simulink model "SP_OEL2"  (R2023b)
settings: Solver=ode23t  StartTime=0.0  StopTime=0.6  MaxStep=simulation.maxStepSize  RelTol=1e-3  AbsTol=1e-3
PostLoadFcn:
  | run('OCR_input.m');
  | run('OCR_settings.m');
InitFcn:
  | run('OCR_settings.m');
undefined symbols (not defined in the file or in its folder): relay1, relay2, source
libraries: ee_lib x14, fl_lib x8, eeGeneralControl x8, simulink x4, simulink_extras x4, nesl_utility x2
(part 1 of 2)
CloseFcn:
  | try, close(h1_ee_relay_overcurrent_phase), end
  | clear h1_ee_relay_overcurrent_phase
  | try, close(h2_ee_relay_overcurrent_earth), end
  | clear h2_ee_relay_overcurrent_earth
  | clear source;
  | clear transformer;
  | clear distributionLine1;
  | clear distributionLine2;
  | clear load;
  | clear sensor1;
  | clear sensor2;
  | clear fault;
  | clear protection;
  | clear maskParameter;
  | clear simlog_ee_relay_overcurrent_protection;
  | clear simulation;
  | clear relay1;
  | clear relay2;
  | clear plotVar;
  | clear relayType;
  | clear mask;
Description:
  | Overcurrent Relay Protection in AC Microgrid
settings Model: Creator=The MathWorks, Inc.  LastModifiedBy=hazwani
settings SolverCC: MaxConsecutiveZCs=100000  MaxConsecutiveMinStep=1000  MaxZcPerStep=1
settings DataIOCC: SaveOutput=off  SignalLogging=off  DSMLogging=off  SaveTime=off  ReturnWorkspaceOutputs=off
settings OptimizationCC: ReuseModelBlockBuffer=off
settings DebuggingCC: UnconnectedInputMsg=warning  UnconnectedOutputMsg=warning  UnconnectedLineMsg=warning
settings ModelReferenceCC: EnableRefExpFcnMdlSchedulingChecks=on
settings RTWCC: DLArmComputeVersion=19.05
settings SimscapeCC: SimscapeLogType=all  SimscapeLogName=simlog_ee_relay_overcurrent_protection  SimscapeLogLimitData=off

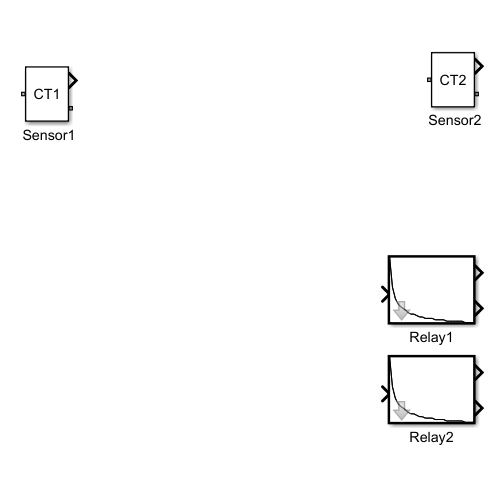
[thumbnail: Simulink's stored preview of the top-level diagram]
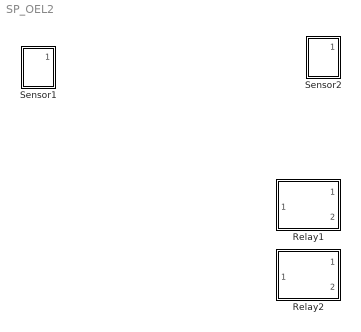
== system SP_OEL2 ==
  " Sensor1" : Subsystem
      mask Display: disp('CT1')
  " Sensor2" : Subsystem
      mask Display: disp('CT2')
  Relay1 : Subsystem  TreatAsAtomicUnit=on  SystemSampleTime=relay1.sampleTime  mask{relayCharacteristicPhase=IEEE Moderately Inverse, relayCharacteristicEarth=IEEE Moderately Inverse, ratedFrequency=source.ratedFrequency, sampleTime=relay1.sampleTime, protectionEnable=1, currentPhase=[1.5 2.5 3.5 4.5 5.5 6.5 7.5 8.5 9.5 10.5], tmsPhase=[0.1 0.2], topPhase=[0.64 1.29;0.29 0.58;0.21 0.43;0.18 0.36;0.16 0.32;0.15 0.29;0.14 0.27;0.13 0.26;0.12 0.25;0.12 0.24], currentEarth=[0.06 0.15 0.2 0.25 0.3 0.35 0.4 0.45 0.5 0.55], tmsEarth=[0.1 0.2], topEarth=[0.64 1.29;0.29 0.58;0.21 0.43;0.18 0.36;0.16 0.32;0.15 0.29;0.14 0.27;0.13 0.26;0.12 0.25;0.12 0.24], phPickUp=relay1.phFltPickUp, ethPickUp=relay1.erFltPickUp, phTimeSetting=relay1.phFltTMS, ethTimeSetting=relay1.erFltTMS, topPhaseActual=0.2, topEarthActual=0.3}
      mask prompts: relayCharacteristicPhase "Relay characteristics for phase protection"; relayCharacteristicEarth "Relay characteristics for earth protection"; ratedFrequency "Fundamental frequency (Hz)"; sampleTime "Relay sample time (s)"; protectionEnable "Relay operation enable"; currentPhase "Current setting for phase protection (A)"; tmsPhase "Time multiplier setting for phase protection (s)"; topPhase "Operating time for phase protection (s)"; currentEarth "Current setting for earth protection (A)"; tmsEarth "Time multiplier setting for earth protection (s)"; topEarth "Operating time for earth protection (s)"; phPickUp "Pick up current for phase protection (A)"; ethPickUp "Pick up current for earth protection (A)"; phTimeSetting "Time multiplier setting for phase protection (s)"; ethTimeSetting "Time multiplier setting for earth protection (s)"; topPhaseActual "Relay operating time for phase protection (s)"; topEarthActual "Relay operating time for earth protection (s)"
      mask TypeOptions relayCharacteristicPhase: IEC Normal Inverse | IEC Very Inverse | IEC Extremely Inverse | IEEE Moderately Inverse | IEEE Very Inverse | IEEE Extremely Inverse | Definite Time | IvsT
      mask Callback relayCharacteristicPhase:
      | % Control parameter visiblity
      | enablePhase = get_param(gcb,'relayCharacteristicPhase');
      | enableEarth = get_param(gcb,'relayCharacteristicEarth');
      | % Set the 'MaskVisibilities' property for each parameters
      | cArray=cell(1,17);
      | cArray(:)={'on'};
      | p=strcmp(enablePhase,'IvsT');
      | q=strcmp(enableEarth,'IvsT');
      | r=strcmp(enablePhase,'Definite Time');
      | s=strcmp(enableEarth,'Definite Time');
      | if p==0 && q==1
      |     cArray(6:8)={'off'};
      | elseif p==0 && q==0
      |     cArray(6:11)={'off'};
      | elseif p==1 && q==0
      |     cArray(9:11)={'off'};
      | end
      | if r==0 && s==1
      |     cArray(15)={'off'};
      |     cArray(16)={'off'};
      | elseif r==0 && s==0
      |     cArray(16:17)={'off'};
      | elseif r==1 && s==0
      |     cArray(14)={'off'};
      |     cArray(17)={'off'};
      | elseif r==1 && s==1
      |     cArray(14:15)={'off'};
      | end
      | set_param(gcb,'MaskVisibilities',cArray);
      mask TypeOptions relayCharacteristicEarth: IEC Normal Inverse | IEC Very Inverse | IEC Extremely Inverse | IEEE Moderately Inverse | IEEE Very Inverse | IEEE Extremely Inverse | Definite Time | IvsT
      mask Callback relayCharacteristicEarth:
      | % Control parameter visiblity
      | enablePhase = get_param(gcb,'relayCharacteristicPhase');
      | enableEarth = get_param(gcb,'relayCharacteristicEarth');
      | % Set the 'MaskVisibilities' property for each parameters
      | cArray=cell(1,17);
      | cArray(:)={'on'};
      | p=strcmp(enablePhase,'IvsT');
      | q=strcmp(enableEarth,'IvsT');
      | r=strcmp(enablePhase,'Definite Time');
      | s=strcmp(enableEarth,'Definite Time');
      | if p==0 && q==1
      |     cArray(6:8)={'off'};
      | elseif p==0 && q==0
      |     cArray(6:11)={'off'};
      | elseif p==1 && q==0
      |     cArray(9:11)={'off'};
      | end
      | if r==0 && s==1
      |     cArray(15)={'off'};
      |     cArray(16)={'off'};
      | elseif r==0 && s==0
      |     cArray(16:17)={'off'};
      | elseif r==1 && s==0
      |     cArray(14)={'off'};
      |     cArray(17)={'off'};
      | elseif r==1 && s==1
      |     cArray(14:15)={'off'};
      | end
      | set_param(gcb,'MaskVisibilities',cArray);
      mask DialogControl Container9 Prompt: Main
      mask DialogControl Container24 Prompt: Current Settings
      mask DialogControl Container19 Prompt: Time Settings
      mask Display:
      | psm = 1:1:30; % Plug setting multiplier
      | tms=0.01; % Time multiplier setting is assumed to be 0.01s
      | top=ones(2,length(psm));  % Operating time of the relay
      | maskParameter=Simulink.Mask.get(gcb); % Get the mask parameters
      | for i=1:2
      |     index(i)=find(strcmp(maskParameter.Parameters(1,i).Value,maskParameter.Parameters(1,i).TypeOptions));
      |     if index(i)<7
      |         switch index(i)              % Selection of relay characteristic
      |             case 1                   % IEC Normal Inverse
      |                 a=0.14;
      |                 b=0.02;
      |                 c=0;
      |             case 2                   % IEC Very Inverse
      |                 a=13.5;
      |                 b=1;
      |                 c=0;
      |             case 3                   % IEC Extremely Inverse
      |                 a=80;
      |                 b=2;
      |                 c=0;
      |             case 4                   % IEEE Moderately Inverse
      |                 a=0.0515;
      |                 b=0.02;
      |                 c=0.114;
      |             case 5                   % IEEE Very Inverse
      |                 a=19.61;
      |                 b=2;
      |                 c=0.491;
      |             otherwise                % IEEE Exteremely Inverse
      |                 a=28.2;
      |                 b=2;
      |                 c=0.1217;
      |         end
      |         for j=1:length(psm)
      |             top(i,j)=tms*((a/(power(psm(j),b)-1))+c); % Operating time of the relay
      |         end
      |     else
      |         top(i,1:length(psm))=0.03*ones(1,length(psm));% Operating time of the relay
      |     end
      | end
      | top1=top(1,1:end);
      | top2=top(2,1:end);
      | 
      | maskFigure=figure;
      | if index(1)<8
      |     plot(psm,top1)
      | else
      |     fprintf('\n\nIvsT');
      | end
      | hold on;
      | if index(2)<8
      |     plot(psm,top2);
      | elseif index(1)<8
      |     fprintf('\nIvsT');
      | end
      | close(maskFigure);
  Relay2 : Subsystem  TreatAsAtomicUnit=on  SystemSampleTime=relay1.sampleTime  mask{relayCharacteristicPhase=IEEE Moderately Inverse, relayCharacteristicEarth=IEEE Moderately Inverse, ratedFrequency=source.ratedFrequency, sampleTime=relay2.sampleTime, protectionEnable=1, currentPhase=[1.5 2.5 3.5 4.5 5.5 6.5 7.5 8.5 9.5 10.5], tmsPhase=[0.1 0.2], topPhase=[0.64 1.29;0.29 0.58;0.21 0.43;0.18 0.36;0.16 0.32;0.15 0.29;0.14 0.27;0.13 0.26;0.12 0.25;0.12 0.24], currentEarth=[0.06 0.15 0.2 0.25 0.3 0.35 0.4 0.45 0.5 0.55], tmsEarth=[0.1 0.2], topEarth=[0.64 1.29;0.29 0.58;0.21 0.43;0.18 0.36;0.16 0.32;0.15 0.29;0.14 0.27;0.13 0.26;0.12 0.25;0.12 0.24], phPickUp=relay2.phFltPickUp, ethPickUp=relay2.erFltPickUp, phTimeSetting=relay2.phFltTMS, ethTimeSetting=relay2.erFltTMS, topPhaseActual=0.2, topEarthActual=0.3}
      mask prompts: relayCharacteristicPhase "Relay characteristics for phase protection"; relayCharacteristicEarth "Relay characteristics for earth protection"; ratedFrequency "Fundamental frequency (Hz)"; sampleTime "Relay sample time (s)"; protectionEnable "Relay operation enable"; currentPhase "Current setting for phase protection (A)"; tmsPhase "Time multiplier setting for phase protection (s)"; topPhase "Operating time for phase protection (s)"; currentEarth "Current setting for earth protection (A)"; tmsEarth "Time multiplier setting for earth protection (s)"; topEarth "Operating time for earth protection (s)"; phPickUp "Pick up current for phase protection (A)"; ethPickUp "Pick up current for earth protection (A)"; phTimeSetting "Time multiplier setting for phase protection (s)"; ethTimeSetting "Time multiplier setting for earth protection (s)"; topPhaseActual "Relay operating time for phase protection (s)"; topEarthActual "Relay operating time for earth protection (s)"
      mask TypeOptions relayCharacteristicPhase: IEC Normal Inverse | IEC Very Inverse | IEC Extremely Inverse | IEEE Moderately Inverse | IEEE Very Inverse | IEEE Extremely Inverse | Definite Time | IvsT
      mask Callback relayCharacteristicPhase:
      | % Control parameter visiblity
      | enablePhase = get_param(gcb,'relayCharacteristicPhase');
      | enableEarth = get_param(gcb,'relayCharacteristicEarth');
      | % Set the 'MaskVisibilities' property for each parameters
      | cArray=cell(1,17);
      | cArray(:)={'on'};
      | p=strcmp(enablePhase,'IvsT');
      | q=strcmp(enableEarth,'IvsT');
      | r=strcmp(enablePhase,'Definite Time');
      | s=strcmp(enableEarth,'Definite Time');
      | if p==0 && q==1
      |     cArray(6:8)={'off'};
      | elseif p==0 && q==0
      |     cArray(6:11)={'off'};
      | elseif p==1 && q==0
      |     cArray(9:11)={'off'};
      | end
      | if r==0 && s==1
      |     cArray(15)={'off'};
      |     cArray(16)={'off'};
      | elseif r==0 && s==0
      |     cArray(16:17)={'off'};
      | elseif r==1 && s==0
      |     cArray(14)={'off'};
      |     cArray(17)={'off'};
      | elseif r==1 && s==1
      |     cArray(14:15)={'off'};
      | end
      | set_param(gcb,'MaskVisibilities',cArray);
      mask TypeOptions relayCharacteristicEarth: IEC Normal Inverse | IEC Very Inverse | IEC Extremely Inverse | IEEE Moderately Inverse | IEEE Very Inverse | IEEE Extremely Inverse | Definite Time | IvsT
      mask Callback relayCharacteristicEarth:
      | % Control parameter visiblity
      | enablePhase = get_param(gcb,'relayCharacteristicPhase');
      | enableEarth = get_param(gcb,'relayCharacteristicEarth');
      | % Set the 'MaskVisibilities' property for each parameters
      | cArray=cell(1,17);
      | cArray(:)={'on'};
      | p=strcmp(enablePhase,'IvsT');
      | q=strcmp(enableEarth,'IvsT');
      | r=strcmp(enablePhase,'Definite Time');
      | s=strcmp(enableEarth,'Definite Time');
      | if p==0 && q==1
      |     cArray(6:8)={'off'};
      | elseif p==0 && q==0
      |     cArray(6:11)={'off'};
      | elseif p==1 && q==0
      |     cArray(9:11)={'off'};
      | end
      | if r==0 && s==1
      |     cArray(15)={'off'};
      |     cArray(16)={'off'};
      | elseif r==0 && s==0
      |     cArray(16:17)={'off'};
      | elseif r==1 && s==0
      |     cArray(14)={'off'};
      |     cArray(17)={'off'};
      | elseif r==1 && s==1
      |     cArray(14:15)={'off'};
      | end
      | set_param(gcb,'MaskVisibilities',cArray);
      mask DialogControl Container9 Prompt: Main
      mask DialogControl Container24 Prompt: Current Settings
      mask DialogControl Container19 Prompt: Time Settings
      mask Display:
      | psm = 1:1:30; % Plug setting multiplier
      | tms=0.01; % Time multiplier setting is assumed to be 0.01s
      | top=ones(2,length(psm));  % Operating time of the relay
      | maskParameter=Simulink.Mask.get(gcb); % Get the mask parameters
      | for i=1:2
      |     index(i)=find(strcmp(maskParameter.Parameters(1,i).Value,maskParameter.Parameters(1,i).TypeOptions));
      |     if index(i)<7
      |         switch index(i)              % Selection of relay characteristic
      |             case 1                   % IEC Normal Inverse
      |                 a=0.14;
      |                 b=0.02;
      |                 c=0;
      |             case 2                   % IEC Very Inverse
      |                 a=13.5;
      |                 b=1;
      |                 c=0;
      |             case 3                   % IEC Extremely Inverse
      |                 a=80;
      |                 b=2;
      |                 c=0;
      |             case 4                   % IEEE Moderately Inverse
      |                 a=0.0515;
      |                 b=0.02;
      |                 c=0.114;
      |             case 5                   % IEEE Very Inverse
      |                 a=19.61;
      |                 b=2;
      |                 c=0.491;
      |             otherwise                % IEEE Exteremely Inverse
      |                 a=28.2;
      |                 b=2;
      |                 c=0.1217;
      |         end
      |         for j=1:length(psm)
      |             top(i,j)=tms*((a/(power(psm(j),b)-1))+c); % Operating time of the relay
      |         end
      |     else
      |         top(i,1:length(psm))=0.03*ones(1,length(psm));% Operating time of the relay
      |     end
      | end
      | top1=top(1,1:end);
      | top2=top(2,1:end);
      | 
      | maskFigure=figure;
      | if index(1)<8
      |     plot(psm,top1)
      | else
      |     fprintf('\n\nIvsT');
      | end
      | hold on;
      | if index(2)<8
      |     plot(psm,top2);
      | elseif index(1)<8
      |     fprintf('\nIvsT');
      | end
      | close(maskFigure);

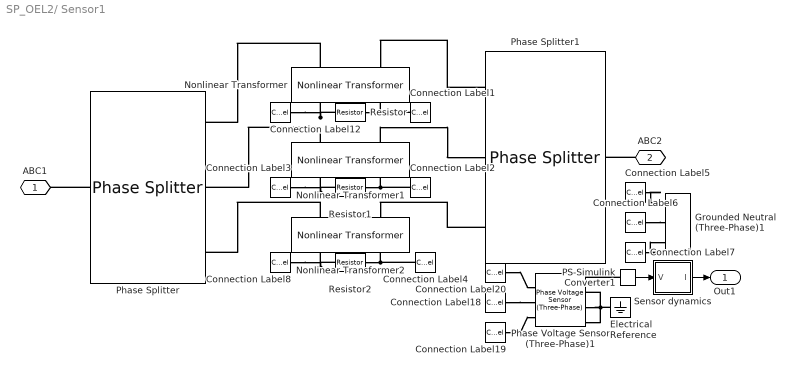
== system SP_OEL2/ Sensor1 ==
  Connection Label1 : ConnectionLabel  Label=Ian
  Connection Label12 : ConnectionLabel  Label=Iap
  Connection Label18 : ConnectionLabel  Label=Ibp
  Connection Label19 : ConnectionLabel  Label=Icp
  Connection Label2 : ConnectionLabel  Label=Ibn
  Connection Label20 : ConnectionLabel  Label=Iap
  Connection Label3 : ConnectionLabel  Label=Ibp
  Connection Label4 : ConnectionLabel  Label=Ibn
  Connection Label5 : ConnectionLabel  Label=Ian
  Connection Label6 : ConnectionLabel  Label=Ibn
  Connection Label7 : ConnectionLabel  Label=Icn
  Connection Label8 : ConnectionLabel  Label=Icp
  Electrical Reference : fl_lib/Electrical/Electrical Elements/Electrical Reference
  Grounded Neutral (Three-Phase)1 : ee_lib/Connectors & References/Grounded Neutral (Three-Phase)
      settings: InternalSimscapePortConfiguration="{\"Bottom\":[],\"Left\":[{\"id\":\"a\",\"label\":\"a\",\"type\":\"foundation.electrical.electrical\"},{\"id\":\"b\",\"label\":\"b\",\"type\":\"foundation.electrical.electrical\"},{\"id\":\"c\",\"label\":\"c\",\"type\":\"foundation.electrical.electrical\"}],\"Right\":[],\"Top\":[]}"
  Nonlinear Transformer : ee_lib/Passive/Transformers/Nonlinear Transformer  Nw=1  Nw2=sensor1.ctRatio  winding_param_option=1  Req=1e-3 Ohm  Leq=1e-4 H  R_1=0.01 Ohm  L_1=0.0001 H  R_2=0.01 Ohm  L_2=0.0001 H  averaging_period=0 s  R_m=100 Ohm  parameterization_option=1  H_data=[0, 200, 400, 600, 800, 1000] A/m  B_data=[0, .81, 1.25, 1.42, 1.48, 1.49] T  length_effective=0.2 m  area_effective=2e-4 m^2  L=4e-2 H  L_sat=1e-2 H  current_data=[0, .4, .8, 1.2, 1.6, 2] A  magnetic_flux_data=[0, .161, .25, .284, .295, .299] .* 1e-3 Wb  magnetic_flux_sat=1.6e-04 Wb  dBdH0=0.005 m*T/A  B1=1.49 T  H1=1000 A/m  c=0.1  K=200 A/m  alpha=1e-4  interpolation_option=1  Leq_i0=0 A  L1_i0=0 A  L2_i0=0 A  x0_option=1  i_L0=0 A  phi0=0 Wb  B0=0 T  H0=0 A/m  Leq_g=1e-9 1/Ohm  L1_g=1e-9 1/Ohm  L2_g=1e-9 1/Ohm
      settings: InternalSimscapePortConfiguration="{\"Bottom\":[],\"Left\":[{\"id\":\"p1\",\"label\":\"1+\",\"type\":\"foundation.electrical.electrical\"},{\"id\":\"n1\",\"label\":\"1-\",\"type\":\"foundation.electrical.electrical\"}],\"Right\":[{\"id\":\"p2\",\"label\":\"2+\",\"type\":\"foundation.electrical.electrical\"},{\"id\":\"n2\",\"label\":\"2-\",\"type\":\"foundation.electrical.electrical\"}],\"Top\":[]}"
  Nonlinear Transformer1 : ee_lib/Passive/Transformers/Nonlinear Transformer  Nw=1  Nw2=sensor1.ctRatio  winding_param_option=1  Req=1e-3 Ohm  Leq=1e-4 H  R_1=0.01 Ohm  L_1=0.0001 H  R_2=0.01 Ohm  L_2=0.0001 H  averaging_period=0 s  R_m=100 Ohm  parameterization_option=1  H_data=[0, 200, 400, 600, 800, 1000] A/m  B_data=[0, .81, 1.25, 1.42, 1.48, 1.49] T  length_effective=0.2 m  area_effective=2e-4 m^2  L=4e-2 H  L_sat=1e-2 H  current_data=[0, .4, .8, 1.2, 1.6, 2] A  magnetic_flux_data=[0, .161, .25, .284, .295, .299] .* 1e-3 Wb  magnetic_flux_sat=1.6e-04 Wb  dBdH0=0.005 m*T/A  B1=1.49 T  H1=1000 A/m  c=0.1  K=200 A/m  alpha=1e-4  interpolation_option=1  Leq_i0=0 A  L1_i0=0 A  L2_i0=0 A  x0_option=1  i_L0=0 A  phi0=0 Wb  B0=0 T  H0=0 A/m  Leq_g=1e-9 1/Ohm  L1_g=1e-9 1/Ohm  L2_g=1e-9 1/Ohm
      settings: InternalSimscapePortConfiguration="{\"Bottom\":[],\"Left\":[{\"id\":\"p1\",\"label\":\"1+\",\"type\":\"foundation.electrical.electrical\"},{\"id\":\"n1\",\"label\":\"1-\",\"type\":\"foundation.electrical.electrical\"}],\"Right\":[{\"id\":\"p2\",\"label\":\"2+\",\"type\":\"foundation.electrical.electrical\"},{\"id\":\"n2\",\"label\":\"2-\",\"type\":\"foundation.electrical.electrical\"}],\"Top\":[]}"
  Nonlinear Transformer2 : ee_lib/Passive/Transformers/Nonlinear Transformer  Nw=1  Nw2=sensor1.ctRatio  winding_param_option=1  Req=1e-3 Ohm  Leq=1e-4 H  R_1=0.01 Ohm  L_1=0.0001 H  R_2=0.01 Ohm  L_2=0.0001 H  averaging_period=0 s  R_m=100 Ohm  parameterization_option=1  H_data=[0, 200, 400, 600, 800, 1000] A/m  B_data=[0, .81, 1.25, 1.42, 1.48, 1.49] T  length_effective=0.2 m  area_effective=2e-4 m^2  L=4e-2 H  L_sat=1e-2 H  current_data=[0, .4, .8, 1.2, 1.6, 2] A  magnetic_flux_data=[0, .161, .25, .284, .295, .299] .* 1e-3 Wb  magnetic_flux_sat=1.6e-04 Wb  dBdH0=0.005 m*T/A  B1=1.49 T  H1=1000 A/m  c=0.1  K=200 A/m  alpha=1e-4  interpolation_option=1  Leq_i0=0 A  L1_i0=0 A  L2_i0=0 A  x0_option=1  i_L0=0 A  phi0=0 Wb  B0=0 T  H0=0 A/m  Leq_g=1e-9 1/Ohm  L1_g=1e-9 1/Ohm  L2_g=1e-9 1/Ohm
      settings: InternalSimscapePortConfiguration="{\"Bottom\":[],\"Left\":[{\"id\":\"p1\",\"label\":\"1+\",\"type\":\"foundation.electrical.electrical\"},{\"id\":\"n1\",\"label\":\"1-\",\"type\":\"foundation.electrical.electrical\"}],\"Right\":[{\"id\":\"p2\",\"label\":\"2+\",\"type\":\"foundation.electrical.electrical\"},{\"id\":\"n2\",\"label\":\"2-\",\"type\":\"foundation.electrical.electrical\"}],\"Top\":[]}"
  PS-Simulink Converter1 : nesl_utility/PS-Simulink Converter  PhysicalDomain=network_engine_domain  SubClassName=ps_output  LeftPortType=input  RightPortType=output  PseudoPeriodic=off  Frequencies=[]  VectorFormat=1-D array  Unit=inherit  AffineConversion=off
  Phase Splitter : ee_lib/Connectors & References/Phase Splitter
  Phase Splitter1 : ee_lib/Connectors & References/Phase Splitter
  Phase Voltage Sensor (Three-Phase)1 : ee_lib/Sensors & Transducers/Phase Voltage Sensor (Three-Phase)
      settings: LogSimulationData=on  InternalSimscapePortConfiguration="{\"Bottom\":[],\"Left\":[{\"id\":\"a1\",\"label\":\"a1\",\"type\":\"foundation.electrical.electrical\"},{\"id\":\"b1\",\"label\":\"b1\",\"type\":\"foundation.electrical.electrical\"},{\"id\":\"c1\",\"label\":\"c1\",\"type\":\"foundation.electrical.electrical\"}],\"Right\":[{\"id\":\"V_output\",\"label\":\"V\",\"type\":\"output\"},{\"id\":\"a2\",\"label\":\"a2\",\"type\":\"foundation.electrical.electrical\"},{\"id\":\"b2\",\"label\":\"b2\",\"type\":\"foundation.electrical.electrical\"},{\"id\":\"c2\",\"label\":\"c2\",\"type\":\"foundation.electrical.electrical\"}],\"Top\":[]}"
  Resistor : fl_lib/Electrical/Electrical Elements/Resistor  R=1 Ohm  i_specify=off  i_priority=None  i=0 A  i_nominal_specify=off  i_nominal_unit=A  i_nominal_value=1  v_specify=off  v_priority=None  v=0 V  v_nominal_specify=off  v_nominal_unit=V  v_nominal_value=1
  Resistor1 : fl_lib/Electrical/Electrical Elements/Resistor  R=1 Ohm  i_specify=off  i_priority=None  i=0 A  i_nominal_specify=off  i_nominal_unit=A  i_nominal_value=1  v_specify=off  v_priority=None  v=0 V  v_nominal_specify=off  v_nominal_unit=V  v_nominal_value=1
  Resistor2 : fl_lib/Electrical/Electrical Elements/Resistor  R=1 Ohm  i_specify=off  i_priority=None  i=0 A  i_nominal_specify=off  i_nominal_unit=A  i_nominal_value=1  v_specify=off  v_priority=None  v=0 V  v_nominal_specify=off  v_nominal_unit=V  v_nominal_value=1
  Sensor dynamics : Subsystem
  ABC1 : PMIOPort  Side=Left
  ABC2 : PMIOPort  Port=2  Side=Right
  Out1 : Outport
  wires:
  PS-Simulink Converter1/1 -> Sensor dynamics/1(V)
  Sensor dynamics/1(I) -> Out1/1
  connections:
  Phase Splitter/LConn1 -- ABC1/RConn1
  ABC2/RConn1 -- Phase Splitter1/LConn1
  Connection Label19/LConn1 -- Phase Voltage Sensor (Three-Phase)1/LConn3
  Connection Label18/LConn1 -- Phase Voltage Sensor (Three-Phase)1/LConn2
  PS-Simulink Converter1/LConn1 -- Phase Voltage Sensor (Three-Phase)1/RConn1
  Connection Label20/LConn1 -- Phase Voltage Sensor (Three-Phase)1/LConn1
  Nonlinear Transformer/RConn1 -- Resistor/LConn1 -- Connection Label12/LConn1
  Nonlinear Transformer/LConn1 -- Phase Splitter/RConn1
  Phase Splitter1/RConn1 -- Nonlinear Transformer/LConn2
  Resistor/RConn1 -- Connection Label1/LConn1 -- Nonlinear Transformer/RConn2
  Nonlinear Transformer1/RConn1 -- Resistor1/LConn1 -- Connection Label3/LConn1
  Nonlinear Transformer1/LConn2 -- Phase Splitter1/RConn2
  Nonlinear Transformer1/LConn1 -- Phase Splitter/RConn2
  Nonlinear Transformer2/RConn1 -- Resistor2/LConn1 -- Connection Label8/LConn1
  Nonlinear Transformer2/LConn1 -- Phase Splitter/RConn3
  Phase Splitter1/RConn3 -- Nonlinear Transformer2/LConn2
  Resistor2/RConn1 -- Connection Label4/LConn1 -- Nonlinear Transformer2/RConn2
  Resistor1/RConn1 -- Nonlinear Transformer1/RConn2 -- Connection Label2/LConn1
  Electrical Reference/LConn1 -- Phase Voltage Sensor (Three-Phase)1/RConn2 -- Phase Voltage Sensor (Three-Phase)1/RConn3 -- Phase Voltage Sensor (Three-Phase)1/RConn4
  Connection Label5/LConn1 -- Grounded Neutral (Three-Phase)1/LConn1
  Connection Label6/LConn1 -- Grounded Neutral (Three-Phase)1/LConn2
  Connection Label7/LConn1 -- Grounded Neutral (Three-Phase)1/LConn3

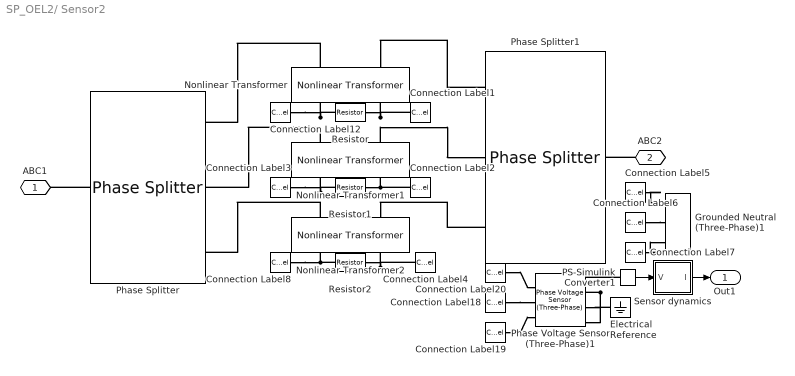
== system SP_OEL2/ Sensor2 ==
  Connection Label1 : ConnectionLabel  Label=Ian
  Connection Label12 : ConnectionLabel  Label=Iap
  Connection Label18 : ConnectionLabel  Label=Ibp
  Connection Label19 : ConnectionLabel  Label=Icp
  Connection Label2 : ConnectionLabel  Label=Ibn
  Connection Label20 : ConnectionLabel  Label=Iap
  Connection Label3 : ConnectionLabel  Label=Ibp
  Connection Label4 : ConnectionLabel  Label=Ibn
  Connection Label5 : ConnectionLabel  Label=Ian
  Connection Label6 : ConnectionLabel  Label=Ibn
  Connection Label7 : ConnectionLabel  Label=Icn
  Connection Label8 : ConnectionLabel  Label=Icp
  Electrical Reference : fl_lib/Electrical/Electrical Elements/Electrical Reference
  Grounded Neutral (Three-Phase)1 : ee_lib/Connectors & References/Grounded Neutral (Three-Phase)
      settings: InternalSimscapePortConfiguration="{\"Bottom\":[],\"Left\":[{\"id\":\"a\",\"label\":\"a\",\"type\":\"foundation.electrical.electrical\"},{\"id\":\"b\",\"label\":\"b\",\"type\":\"foundation.electrical.electrical\"},{\"id\":\"c\",\"label\":\"c\",\"type\":\"foundation.electrical.electrical\"}],\"Right\":[],\"Top\":[]}"
  Nonlinear Transformer : ee_lib/Passive/Transformers/Nonlinear Transformer  Nw=1  Nw2=sensor2.ctRatio  winding_param_option=1  Req=1e-3 Ohm  Leq=1e-4 H  R_1=0.01 Ohm  L_1=0.0001 H  R_2=0.01 Ohm  L_2=0.0001 H  averaging_period=0 s  R_m=100 Ohm  parameterization_option=1  H_data=[0, 200, 400, 600, 800, 1000] A/m  B_data=[0, .81, 1.25, 1.42, 1.48, 1.49] T  length_effective=0.2 m  area_effective=2e-4 m^2  L=4e-2 H  L_sat=1e-2 H  current_data=[0, .4, .8, 1.2, 1.6, 2] A  magnetic_flux_data=[0, .161, .25, .284, .295, .299] .* 1e-3 Wb  magnetic_flux_sat=1.6e-04 Wb  dBdH0=0.005 m*T/A  B1=1.49 T  H1=1000 A/m  c=0.1  K=200 A/m  alpha=1e-4  interpolation_option=1  Leq_i0=0 A  L1_i0=0 A  L2_i0=0 A  x0_option=1  i_L0=0 A  phi0=0 Wb  B0=0 T  H0=0 A/m  Leq_g=1e-9 1/Ohm  L1_g=1e-9 1/Ohm  L2_g=1e-9 1/Ohm
      settings: InternalSimscapePortConfiguration="{\"Bottom\":[],\"Left\":[{\"id\":\"p1\",\"label\":\"1+\",\"type\":\"foundation.electrical.electrical\"},{\"id\":\"n1\",\"label\":\"1-\",\"type\":\"foundation.electrical.electrical\"}],\"Right\":[{\"id\":\"p2\",\"label\":\"2+\",\"type\":\"foundation.electrical.electrical\"},{\"id\":\"n2\",\"label\":\"2-\",\"type\":\"foundation.electrical.electrical\"}],\"Top\":[]}"
  Nonlinear Transformer1 : ee_lib/Passive/Transformers/Nonlinear Transformer  Nw=1  Nw2=sensor2.ctRatio  winding_param_option=1  Req=1e-3 Ohm  Leq=1e-4 H  R_1=0.01 Ohm  L_1=0.0001 H  R_2=0.01 Ohm  L_2=0.0001 H  averaging_period=0 s  R_m=100 Ohm  parameterization_option=1  H_data=[0, 200, 400, 600, 800, 1000] A/m  B_data=[0, .81, 1.25, 1.42, 1.48, 1.49] T  length_effective=0.2 m  area_effective=2e-4 m^2  L=4e-2 H  L_sat=1e-2 H  current_data=[0, .4, .8, 1.2, 1.6, 2] A  magnetic_flux_data=[0, .161, .25, .284, .295, .299] .* 1e-3 Wb  magnetic_flux_sat=1.6e-04 Wb  dBdH0=0.005 m*T/A  B1=1.49 T  H1=1000 A/m  c=0.1  K=200 A/m  alpha=1e-4  interpolation_option=1  Leq_i0=0 A  L1_i0=0 A  L2_i0=0 A  x0_option=1  i_L0=0 A  phi0=0 Wb  B0=0 T  H0=0 A/m  Leq_g=1e-9 1/Ohm  L1_g=1e-9 1/Ohm  L2_g=1e-9 1/Ohm
      settings: InternalSimscapePortConfiguration="{\"Bottom\":[],\"Left\":[{\"id\":\"p1\",\"label\":\"1+\",\"type\":\"foundation.electrical.electrical\"},{\"id\":\"n1\",\"label\":\"1-\",\"type\":\"foundation.electrical.electrical\"}],\"Right\":[{\"id\":\"p2\",\"label\":\"2+\",\"type\":\"foundation.electrical.electrical\"},{\"id\":\"n2\",\"label\":\"2-\",\"type\":\"foundation.electrical.electrical\"}],\"Top\":[]}"
  Nonlinear Transformer2 : ee_lib/Passive/Transformers/Nonlinear Transformer  Nw=1  Nw2=sensor2.ctRatio  winding_param_option=1  Req=1e-3 Ohm  Leq=1e-4 H  R_1=0.01 Ohm  L_1=0.0001 H  R_2=0.01 Ohm  L_2=0.0001 H  averaging_period=0 s  R_m=100 Ohm  parameterization_option=1  H_data=[0, 200, 400, 600, 800, 1000] A/m  B_data=[0, .81, 1.25, 1.42, 1.48, 1.49] T  length_effective=0.2 m  area_effective=2e-4 m^2  L=4e-2 H  L_sat=1e-2 H  current_data=[0, .4, .8, 1.2, 1.6, 2] A  magnetic_flux_data=[0, .161, .25, .284, .295, .299] .* 1e-3 Wb  magnetic_flux_sat=1.6e-04 Wb  dBdH0=0.005 m*T/A  B1=1.49 T  H1=1000 A/m  c=0.1  K=200 A/m  alpha=1e-4  interpolation_option=1  Leq_i0=0 A  L1_i0=0 A  L2_i0=0 A  x0_option=1  i_L0=0 A  phi0=0 Wb  B0=0 T  H0=0 A/m  Leq_g=1e-9 1/Ohm  L1_g=1e-9 1/Ohm  L2_g=1e-9 1/Ohm
      settings: InternalSimscapePortConfiguration="{\"Bottom\":[],\"Left\":[{\"id\":\"p1\",\"label\":\"1+\",\"type\":\"foundation.electrical.electrical\"},{\"id\":\"n1\",\"label\":\"1-\",\"type\":\"foundation.electrical.electrical\"}],\"Right\":[{\"id\":\"p2\",\"label\":\"2+\",\"type\":\"foundation.electrical.electrical\"},{\"id\":\"n2\",\"label\":\"2-\",\"type\":\"foundation.electrical.electrical\"}],\"Top\":[]}"
  PS-Simulink Converter1 : nesl_utility/PS-Simulink Converter  PhysicalDomain=network_engine_domain  SubClassName=ps_output  LeftPortType=input  RightPortType=output  PseudoPeriodic=off  Frequencies=[]  VectorFormat=1-D array  Unit=inherit  AffineConversion=off
  Phase Splitter : ee_lib/Connectors & References/Phase Splitter
  Phase Splitter1 : ee_lib/Connectors & References/Phase Splitter
  Phase Voltage Sensor (Three-Phase)1 : ee_lib/Sensors & Transducers/Phase Voltage Sensor (Three-Phase)
      settings: LogSimulationData=on  InternalSimscapePortConfiguration="{\"Bottom\":[],\"Left\":[{\"id\":\"a1\",\"label\":\"a1\",\"type\":\"foundation.electrical.electrical\"},{\"id\":\"b1\",\"label\":\"b1\",\"type\":\"foundation.electrical.electrical\"},{\"id\":\"c1\",\"label\":\"c1\",\"type\":\"foundation.electrical.electrical\"}],\"Right\":[{\"id\":\"V_output\",\"label\":\"V\",\"type\":\"output\"},{\"id\":\"a2\",\"label\":\"a2\",\"type\":\"foundation.electrical.electrical\"},{\"id\":\"b2\",\"label\":\"b2\",\"type\":\"foundation.electrical.electrical\"},{\"id\":\"c2\",\"label\":\"c2\",\"type\":\"foundation.electrical.electrical\"}],\"Top\":[]}"
  Resistor : fl_lib/Electrical/Electrical Elements/Resistor  R=1 Ohm  i_specify=off  i_priority=None  i=0 A  i_nominal_specify=off  i_nominal_unit=A  i_nominal_value=1  v_specify=off  v_priority=None  v=0 V  v_nominal_specify=off  v_nominal_unit=V  v_nominal_value=1
  Resistor1 : fl_lib/Electrical/Electrical Elements/Resistor  R=1 Ohm  i_specify=off  i_priority=None  i=0 A  i_nominal_specify=off  i_nominal_unit=A  i_nominal_value=1  v_specify=off  v_priority=None  v=0 V  v_nominal_specify=off  v_nominal_unit=V  v_nominal_value=1
  Resistor2 : fl_lib/Electrical/Electrical Elements/Resistor  R=1 Ohm  i_specify=off  i_priority=None  i=0 A  i_nominal_specify=off  i_nominal_unit=A  i_nominal_value=1  v_specify=off  v_priority=None  v=0 V  v_nominal_specify=off  v_nominal_unit=V  v_nominal_value=1
  Sensor dynamics : Subsystem
  ABC1 : PMIOPort  Side=Left
  ABC2 : PMIOPort  Port=2  Side=Right
  Out1 : Outport
  wires:
  PS-Simulink Converter1/1 -> Sensor dynamics/1(V)
  Sensor dynamics/1(I) -> Out1/1
  connections:
  Phase Splitter/LConn1 -- ABC1/RConn1
  ABC2/RConn1 -- Phase Splitter1/LConn1
  Connection Label19/LConn1 -- Phase Voltage Sensor (Three-Phase)1/LConn3
  Connection Label18/LConn1 -- Phase Voltage Sensor (Three-Phase)1/LConn2
  PS-Simulink Converter1/LConn1 -- Phase Voltage Sensor (Three-Phase)1/RConn1
  Connection Label20/LConn1 -- Phase Voltage Sensor (Three-Phase)1/LConn1
  Nonlinear Transformer/RConn1 -- Resistor/LConn1 -- Connection Label12/LConn1
  Nonlinear Transformer/LConn1 -- Phase Splitter/RConn1
  Phase Splitter1/RConn1 -- Nonlinear Transformer/LConn2
  Nonlinear Transformer/RConn2 -- Resistor/RConn1 -- Connection Label1/LConn1
  Nonlinear Transformer1/RConn1 -- Resistor1/LConn1 -- Connection Label3/LConn1
  Nonlinear Transformer1/LConn2 -- Phase Splitter1/RConn2
  Nonlinear Transformer1/LConn1 -- Phase Splitter/RConn2
  Resistor2/LConn1 -- Nonlinear Transformer2/RConn1 -- Connection Label8/LConn1
  Nonlinear Transformer2/LConn1 -- Phase Splitter/RConn3
  Phase Splitter1/RConn3 -- Nonlinear Transformer2/LConn2
  Nonlinear Transformer2/RConn2 -- Resistor2/RConn1 -- Connection Label4/LConn1
  Connection Label2/LConn1 -- Resistor1/RConn1 -- Nonlinear Transformer1/RConn2
  Phase Voltage Sensor (Three-Phase)1/RConn2 -- Phase Voltage Sensor (Three-Phase)1/RConn3 -- Electrical Reference/LConn1 -- Phase Voltage Sensor (Three-Phase)1/RConn4
  Connection Label5/LConn1 -- Grounded Neutral (Three-Phase)1/LConn1
  Connection Label6/LConn1 -- Grounded Neutral (Three-Phase)1/LConn2
  Connection Label7/LConn1 -- Grounded Neutral (Three-Phase)1/LConn3

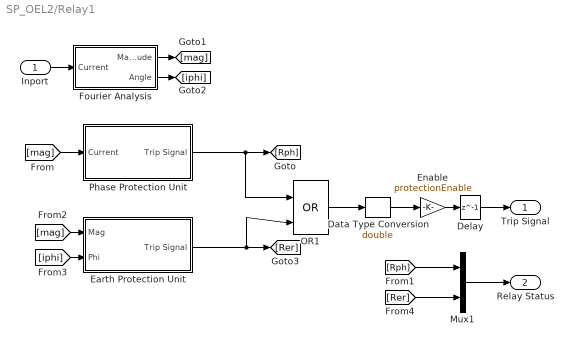
== system SP_OEL2/Relay1 ==
  Inport : Inport
  Data Type Conversion : DataTypeConversion  OutDataTypeStr=double  SaturateOnIntegerOverflow=off  RndMeth=Floor
  Delay : Delay  DelayLength=1
  Earth Protection Unit : Subsystem
  Enable : Gain  Gain=protectionEnable
  Fourier Analysis : Subsystem
  Mux1 : Mux  Inputs=2
  OR1 : Logic  Operator=OR  IconShape=distinctive  AllPortsSameDT=off  OutDataTypeStr=boolean
  Phase Protection Unit : Subsystem
  Trip Signal : Outport
  Relay Status : Outport  Port=2
  wires:
  Data Type Conversion/1 -> Enable/1
  Enable/1 -> Delay/1
  Delay/1 -> Trip Signal/1
  [Rer] -> Mux1/2
  [Rph] -> Mux1/1
  Mux1/1 -> Relay Status/1
  OR1/1 -> Data Type Conversion/1
  Inport/1 -> Fourier Analysis/1(Current)
  Fourier Analysis/1(Magnitude) -> [mag]
  Fourier Analysis/2(Angle) -> [iphi]
  [mag] -> Phase Protection Unit/1(Current)
  [mag] -> Earth Protection Unit/1(Mag)
  [iphi] -> Earth Protection Unit/2(Phi)
  Phase Protection Unit/1(Trip Signal) -> OR1/1, [Rph]
  Earth Protection Unit/1(Trip Signal) -> [Rer], OR1/2

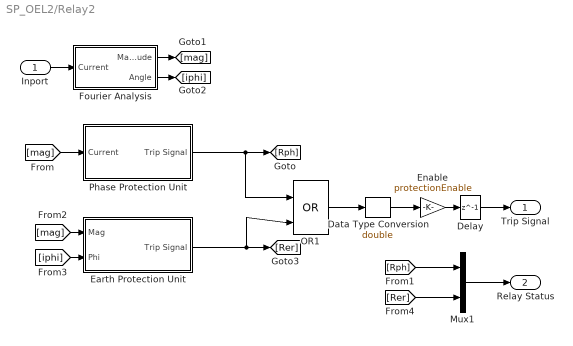
== system SP_OEL2/Relay2 ==
  Inport : Inport
  Data Type Conversion : DataTypeConversion  OutDataTypeStr=double  SaturateOnIntegerOverflow=off  RndMeth=Floor
  Delay : Delay  DelayLength=1
  Earth Protection Unit : Subsystem
  Enable : Gain  Gain=protectionEnable
  Fourier Analysis : Subsystem
  Mux1 : Mux  Inputs=2
  OR1 : Logic  Operator=OR  IconShape=distinctive  AllPortsSameDT=off  OutDataTypeStr=boolean
  Phase Protection Unit : Subsystem
  Trip Signal : Outport
  Relay Status : Outport  Port=2
  wires:
  Data Type Conversion/1 -> Enable/1
  Enable/1 -> Delay/1
  Delay/1 -> Trip Signal/1
  [Rer] -> Mux1/2
  [Rph] -> Mux1/1
  Mux1/1 -> Relay Status/1
  OR1/1 -> Data Type Conversion/1
  Inport/1 -> Fourier Analysis/1(Current)
  Fourier Analysis/1(Magnitude) -> [mag]
  Fourier Analysis/2(Angle) -> [iphi]
  [mag] -> Phase Protection Unit/1(Current)
  [mag] -> Earth Protection Unit/1(Mag)
  [iphi] -> Earth Protection Unit/2(Phi)
  Phase Protection Unit/1(Trip Signal) -> OR1/1, [Rph]
  Earth Protection Unit/1(Trip Signal) -> [Rer], OR1/2

== system SP_OEL2/ Sensor1/Sensor dynamics ==
  V : Inport
  Demux : Demux  Outputs=3
  Mux : Mux  Inputs=3
  Transfer Fcn : TransferFcn  Denominator=[relay1.sampleTime 1]
  Transfer Fcn1 : TransferFcn  Denominator=[relay1.sampleTime 1]
  Transfer Fcn2 : TransferFcn  Denominator=[relay1.sampleTime 1]
  I : Outport
  wires:
  Transfer Fcn/1 -> Mux/1
  Demux/1 -> Transfer Fcn/1
  Demux/3 -> Transfer Fcn2/1
  Mux/1 -> I/1
  Transfer Fcn2/1 -> Mux/3
  Transfer Fcn1/1 -> Mux/2
  Demux/2 -> Transfer Fcn1/1
  V/1 -> Demux/1

== system SP_OEL2/ Sensor2/Sensor dynamics ==
  V : Inport
  Demux : Demux  Outputs=3
  Mux : Mux  Inputs=3
  Transfer Fcn : TransferFcn  Denominator=[relay2.sampleTime 1]
  Transfer Fcn1 : TransferFcn  Denominator=[relay2.sampleTime 1]
  Transfer Fcn2 : TransferFcn  Denominator=[relay2.sampleTime 1]
  I : Outport
  wires:
  Transfer Fcn/1 -> Mux/1
  Demux/1 -> Transfer Fcn/1
  Demux/3 -> Transfer Fcn2/1
  Mux/1 -> I/1
  Transfer Fcn2/1 -> Mux/3
  Transfer Fcn1/1 -> Mux/2
  Demux/2 -> Transfer Fcn1/1
  V/1 -> Demux/1

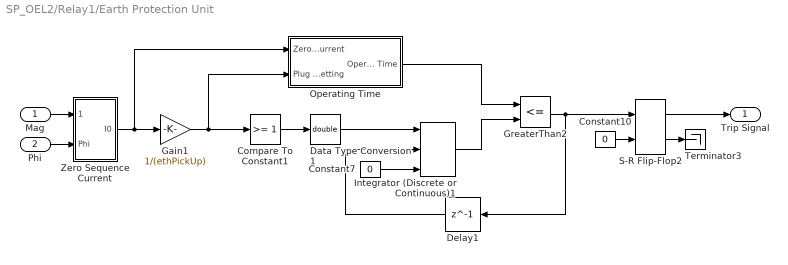
== system SP_OEL2/Relay1/Earth Protection Unit ==
  Mag : Inport
  Phi : Inport  Port=2
  Compare To Constant1 : simulink/Logic and Bit Operations/Compare To Constant  relop=>=  const=1  OutDataTypeStr=boolean
  Constant10 : Constant  Value=0  OutDataTypeStr=boolean
  Constant7 : Constant  Value=0  OutDataTypeStr=double
  Data Type Conversion1 : DataTypeConversion  OutDataTypeStr=double  SaturateOnIntegerOverflow=off  RndMeth=Floor
  Delay1 : Delay  DelayLength=1
  Gain1 : Gain  Gain=1/(ethPickUp)
  GreaterThan2 : RelationalOperator  Operator=<=  OutDataTypeStr=boolean  RndMeth=Simplest  InputSameDT=off
  Integrator (Discrete or Continuous)1 : eeGeneralControl/Integrator (Discrete or Continuous)  LabelModeActiveChoice=Discrete  ExternalReset=falling  LimitType=Anti-windup  B=inf  A=-inf  Ts=sampleTime
  Operating Time : Subsystem
  S-R Flip-Flop2 : simulink_extras/Flip Flops/S-R Flip-Flop  initial_condition=0
  Terminator3 : Terminator
  Zero Sequence Current : Subsystem
  Trip Signal : Outport
  wires:
  Gain1/1 -> Operating Time/2(Plug Setting), Compare To Constant1/1
  Compare To Constant1/1 -> Data Type Conversion1/1
  GreaterThan2/1 -> Delay1/1, S-R Flip-Flop2/1
  Delay1/1 -> Integrator (Discrete or Continuous)1/2
  Constant10/1 -> S-R Flip-Flop2/2
  Zero Sequence Current/1(I0) -> Gain1/1, Operating Time/1(Zero Sequence Current)
  Data Type Conversion1/1 -> Integrator (Discrete or Continuous)1/1
  Integrator (Discrete or Continuous)1/1 -> GreaterThan2/2
  Operating Time/1(Operating Time) -> GreaterThan2/1
  S-R Flip-Flop2/2 -> Terminator3/1
  Constant7/1 -> Integrator (Discrete or Continuous)1/3
  Phi/1 -> Zero Sequence Current/2(Phi)
  Mag/1 -> Zero Sequence Current/1(Mag)
  S-R Flip-Flop2/1 -> Trip Signal/1

== system SP_OEL2/Relay1/Fourier Analysis ==
  Current : Inport
  Add1 : Sum  Inputs=-+
  Delay3 : Delay  DelayLength=1
  Fourier Analysis2 : eeGeneralControl/Fourier Analysis  f=ratedFrequency  n=[1]  M0=0  Ph0=0  BufferSize=8192  Ts=sampleTime
  Gain : Gain  Gain=1/sqrt(2)
  Moving Average : eeGeneralControl/Moving Average  VariantControl=Variant1  LabelModeActiveChoice=Discrete  f=50  x0=0  BufferSize=8192  Ts=sampleTime
  Magnitude : Outport
  Angle : Outport  Port=2
  wires:
  Delay3/1 -> Add1/2, Moving Average/1
  Current/1 -> Delay3/1
  Fourier Analysis2/2 -> Angle/1
  Moving Average/1 -> Add1/1
  Add1/1 -> Fourier Analysis2/1
  Fourier Analysis2/1 -> Gain/1
  Gain/1 -> Magnitude/1

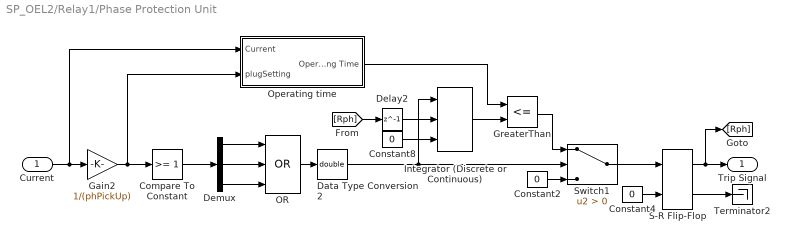
== system SP_OEL2/Relay1/Phase Protection Unit ==
  Current : Inport
  Compare To Constant : simulink/Logic and Bit Operations/Compare To Constant  relop=>=  const=1  OutDataTypeStr=boolean
  Constant2 : Constant  Value=0  OutDataTypeStr=boolean
  Constant4 : Constant  Value=0  OutDataTypeStr=boolean
  Constant8 : Constant  Value=0  OutDataTypeStr=double
  Data Type Conversion2 : DataTypeConversion  OutDataTypeStr=double  SaturateOnIntegerOverflow=off  RndMeth=Floor
  Delay2 : Delay  DelayLength=1
  Demux : Demux  Outputs=3
  Gain2 : Gain  Gain=1/(phPickUp)
  GreaterThan : RelationalOperator  Operator=<=  OutDataTypeStr=boolean  RndMeth=Simplest  InputSameDT=off
  Integrator (Discrete or Continuous) : eeGeneralControl/Integrator (Discrete or Continuous)  LabelModeActiveChoice=Discrete  ExternalReset=falling  LimitType=Anti-windup  B=inf  A=-inf  Ts=sampleTime
  OR : Logic  Operator=OR  Inputs=3  IconShape=distinctive  AllPortsSameDT=off  OutDataTypeStr=boolean
  "Operating time " : Subsystem
  S-R Flip-Flop : simulink_extras/Flip Flops/S-R Flip-Flop  initial_condition=0
  Switch1 : Switch  Criteria=u2 > Threshold  OutDataTypeStr=boolean  SaturateOnIntegerOverflow=off  InputSameDT=off
  Terminator2 : Terminator
  Trip Signal : Outport
  wires:
  Data Type Conversion2/1 -> Integrator (Discrete or Continuous)/1, Switch1/2
  Gain2/1 -> "Operating time "/2(plugSetting), Compare To Constant/1
  Constant2/1 -> Switch1/3
  Demux/2 -> OR/2
  OR/1 -> Data Type Conversion2/1
  Integrator (Discrete or Continuous)/1 -> GreaterThan/2
  Demux/3 -> OR/3
  Current/1 -> Gain2/1, "Operating time "/1(Current)
  GreaterThan/1 -> Switch1/1
  "Operating time "/1(Operating Time) -> GreaterThan/1
  Constant4/1 -> S-R Flip-Flop/2
  S-R Flip-Flop/2 -> Terminator2/1
  Switch1/1 -> S-R Flip-Flop/1
  Demux/1 -> OR/1
  Constant8/1 -> Integrator (Discrete or Continuous)/3
  Compare To Constant/1 -> Demux/1
  S-R Flip-Flop/1 -> Trip Signal/1, [Rph]
  Delay2/1 -> Integrator (Discrete or Continuous)/2
  [Rph] -> Delay2/1

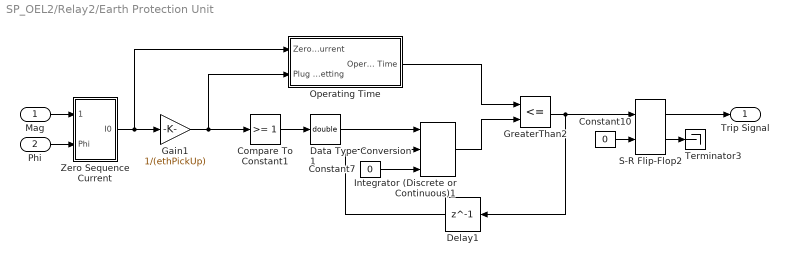
== system SP_OEL2/Relay2/Earth Protection Unit ==
  Mag : Inport
  Phi : Inport  Port=2
  Compare To Constant1 : simulink/Logic and Bit Operations/Compare To Constant  relop=>=  const=1  OutDataTypeStr=boolean
  Constant10 : Constant  Value=0  OutDataTypeStr=boolean
  Constant7 : Constant  Value=0  OutDataTypeStr=double
  Data Type Conversion1 : DataTypeConversion  OutDataTypeStr=double  SaturateOnIntegerOverflow=off  RndMeth=Floor
  Delay1 : Delay  DelayLength=1
  Gain1 : Gain  Gain=1/(ethPickUp)
  GreaterThan2 : RelationalOperator  Operator=<=  OutDataTypeStr=boolean  RndMeth=Simplest  InputSameDT=off
  Integrator (Discrete or Continuous)1 : eeGeneralControl/Integrator (Discrete or Continuous)  LabelModeActiveChoice=Discrete  ExternalReset=falling  LimitType=Anti-windup  B=inf  A=-inf  Ts=sampleTime
  Operating Time : Subsystem
  S-R Flip-Flop2 : simulink_extras/Flip Flops/S-R Flip-Flop  initial_condition=0
  Terminator3 : Terminator
  Zero Sequence Current : Subsystem
  Trip Signal : Outport
  wires:
  Gain1/1 -> Operating Time/2(Plug Setting), Compare To Constant1/1
  Compare To Constant1/1 -> Data Type Conversion1/1
  GreaterThan2/1 -> Delay1/1, S-R Flip-Flop2/1
  Delay1/1 -> Integrator (Discrete or Continuous)1/2
  Constant10/1 -> S-R Flip-Flop2/2
  Zero Sequence Current/1(I0) -> Gain1/1, Operating Time/1(Zero Sequence Current)
  Data Type Conversion1/1 -> Integrator (Discrete or Continuous)1/1
  Integrator (Discrete or Continuous)1/1 -> GreaterThan2/2
  Operating Time/1(Operating Time) -> GreaterThan2/1
  S-R Flip-Flop2/2 -> Terminator3/1
  Constant7/1 -> Integrator (Discrete or Continuous)1/3
  Phi/1 -> Zero Sequence Current/2(Phi)
  Mag/1 -> Zero Sequence Current/1(Mag)
  S-R Flip-Flop2/1 -> Trip Signal/1

== system SP_OEL2/Relay2/Fourier Analysis ==
  Current : Inport
  Add1 : Sum  Inputs=-+
  Delay3 : Delay  DelayLength=1
  Fourier Analysis2 : eeGeneralControl/Fourier Analysis  f=ratedFrequency  n=[1]  M0=0  Ph0=0  BufferSize=8192  Ts=sampleTime
  Gain : Gain  Gain=1/sqrt(2)
  Moving Average : eeGeneralControl/Moving Average  VariantControl=Variant1  LabelModeActiveChoice=Discrete  f=50  x0=0  BufferSize=8192  Ts=sampleTime
  Magnitude : Outport
  Angle : Outport  Port=2
  wires:
  Delay3/1 -> Add1/2, Moving Average/1
  Current/1 -> Delay3/1
  Fourier Analysis2/2 -> Angle/1
  Moving Average/1 -> Add1/1
  Add1/1 -> Fourier Analysis2/1
  Fourier Analysis2/1 -> Gain/1
  Gain/1 -> Magnitude/1

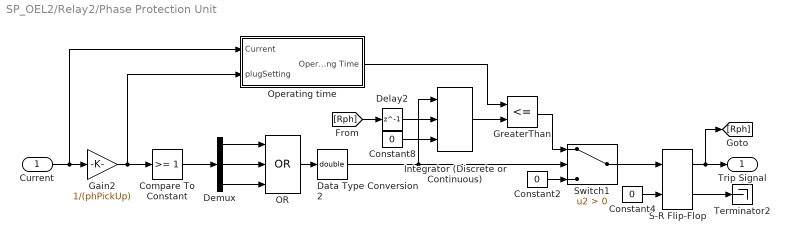
== system SP_OEL2/Relay2/Phase Protection Unit ==
  Current : Inport
  Compare To Constant : simulink/Logic and Bit Operations/Compare To Constant  relop=>=  const=1  OutDataTypeStr=boolean
  Constant2 : Constant  Value=0  OutDataTypeStr=boolean
  Constant4 : Constant  Value=0  OutDataTypeStr=boolean
  Constant8 : Constant  Value=0  OutDataTypeStr=double
  Data Type Conversion2 : DataTypeConversion  OutDataTypeStr=double  SaturateOnIntegerOverflow=off  RndMeth=Floor
  Delay2 : Delay  DelayLength=1
  Demux : Demux  Outputs=3
  Gain2 : Gain  Gain=1/(phPickUp)
  GreaterThan : RelationalOperator  Operator=<=  OutDataTypeStr=boolean  RndMeth=Simplest  InputSameDT=off
  Integrator (Discrete or Continuous) : eeGeneralControl/Integrator (Discrete or Continuous)  LabelModeActiveChoice=Discrete  ExternalReset=falling  LimitType=Anti-windup  B=inf  A=-inf  Ts=sampleTime
  OR : Logic  Operator=OR  Inputs=3  IconShape=distinctive  AllPortsSameDT=off  OutDataTypeStr=boolean
  "Operating time " : Subsystem
  S-R Flip-Flop : simulink_extras/Flip Flops/S-R Flip-Flop  initial_condition=0
  Switch1 : Switch  Criteria=u2 > Threshold  OutDataTypeStr=boolean  SaturateOnIntegerOverflow=off  InputSameDT=off
  Terminator2 : Terminator
  Trip Signal : Outport
  wires:
  Data Type Conversion2/1 -> Integrator (Discrete or Continuous)/1, Switch1/2
  Gain2/1 -> "Operating time "/2(plugSetting), Compare To Constant/1
  Constant2/1 -> Switch1/3
  Demux/2 -> OR/2
  OR/1 -> Data Type Conversion2/1
  Integrator (Discrete or Continuous)/1 -> GreaterThan/2
  Demux/3 -> OR/3
  Current/1 -> Gain2/1, "Operating time "/1(Current)
  GreaterThan/1 -> Switch1/1
  "Operating time "/1(Operating Time) -> GreaterThan/1
  Constant4/1 -> S-R Flip-Flop/2
  S-R Flip-Flop/2 -> Terminator2/1
  Switch1/1 -> S-R Flip-Flop/1
  Demux/1 -> OR/1
  Constant8/1 -> Integrator (Discrete or Continuous)/3
  Compare To Constant/1 -> Demux/1
  S-R Flip-Flop/1 -> Trip Signal/1, [Rph]
  Delay2/1 -> Integrator (Discrete or Continuous)/2
  [Rph] -> Delay2/1

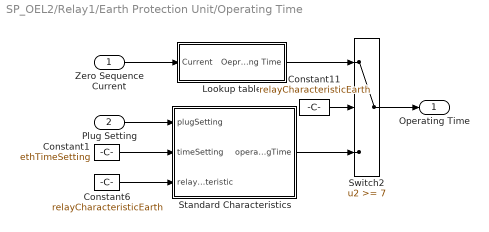
== system SP_OEL2/Relay1/Earth Protection Unit/Operating Time ==
  Zero Sequence Current : Inport
  Plug Setting : Inport  Port=2
  Constant1 : Constant  Value=ethTimeSetting
  Constant11 : Constant  Value=relayCharacteristicEarth
  Constant6 : Constant  Value=relayCharacteristicEarth
  Lookup table : Subsystem
  Standard Characteristics : MATLAB Function  TreatAsAtomicUnit=on
  Switch2 : Switch  Threshold=7  SaturateOnIntegerOverflow=off  InputSameDT=off
  Operating Time : Outport
  wires:
  Constant1/1 -> Standard Characteristics/2(timeSetting)
  Lookup table/1(Oeprating Time) -> Switch2/1
  Constant6/1 -> Standard Characteristics/3(relayCharacteristic)
  Plug Setting/1 -> Standard Characteristics/1(plugSetting)
  Standard Characteristics/1(operatingTime) -> Switch2/3
  Constant11/1 -> Switch2/2
  Switch2/1 -> Operating Time/1
  Zero Sequence Current/1 -> Lookup table/1(Current)

== system SP_OEL2/Relay1/Earth Protection Unit/Zero Sequence Current ==
  Mag : Inport
  Phi : Inport  Port=2
  Add : Sum  Inputs=+++
  Complex to Magnitude-Angle : ComplexToMagnitudeAngle  Output=Magnitude
  Demux1 : Demux  Outputs=3
  Gain : Gain  Gain=1/3
  Magnitude-Angle to Complex : MagnitudeAngleToComplex
  I0 : Outport
  wires:
  Demux1/2 -> Add/2
  Demux1/3 -> Add/3
  Phi/1 -> Magnitude-Angle to Complex/2
  Complex to Magnitude-Angle/1 -> Gain/1
  Demux1/1 -> Add/1
  Mag/1 -> Magnitude-Angle to Complex/1
  Magnitude-Angle to Complex/1 -> Demux1/1
  Add/1 -> Complex to Magnitude-Angle/1
  Gain/1 -> I0/1

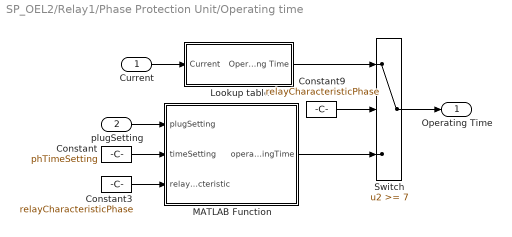
== system SP_OEL2/Relay1/Phase Protection Unit/Operating time  ==
  Current : Inport
  plugSetting : Inport  Port=2
  Constant : Constant  Value=phTimeSetting  VectorParams1D=off
  Constant3 : Constant  Value=relayCharacteristicPhase
  Constant9 : Constant  Value=relayCharacteristicPhase
  "Lookup table " : Subsystem
  MATLAB Function : MATLAB Function  TreatAsAtomicUnit=on
  Switch : Switch  Threshold=7  SaturateOnIntegerOverflow=off  InputSameDT=off
  Operating Time : Outport
  wires:
  Switch/1 -> Operating Time/1
  plugSetting/1 -> MATLAB Function/1(plugSetting)
  Constant9/1 -> Switch/2
  Constant/1 -> MATLAB Function/2(timeSetting)
  Constant3/1 -> MATLAB Function/3(relayCharacteristic)
  MATLAB Function/1(operatingTime) -> Switch/3
  "Lookup table "/1(Operating Time) -> Switch/1
  Current/1 -> "Lookup table "/1(Current)

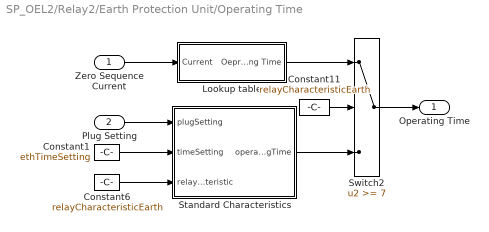
== system SP_OEL2/Relay2/Earth Protection Unit/Operating Time ==
  Zero Sequence Current : Inport
  Plug Setting : Inport  Port=2
  Constant1 : Constant  Value=ethTimeSetting
  Constant11 : Constant  Value=relayCharacteristicEarth
  Constant6 : Constant  Value=relayCharacteristicEarth
  Lookup table : Subsystem
  Standard Characteristics : MATLAB Function  TreatAsAtomicUnit=on
  Switch2 : Switch  Threshold=7  SaturateOnIntegerOverflow=off  InputSameDT=off
  Operating Time : Outport
  wires:
  Constant1/1 -> Standard Characteristics/2(timeSetting)
  Lookup table/1(Oeprating Time) -> Switch2/1
  Constant6/1 -> Standard Characteristics/3(relayCharacteristic)
  Plug Setting/1 -> Standard Characteristics/1(plugSetting)
  Standard Characteristics/1(operatingTime) -> Switch2/3
  Constant11/1 -> Switch2/2
  Switch2/1 -> Operating Time/1
  Zero Sequence Current/1 -> Lookup table/1(Current)

== system SP_OEL2/Relay2/Earth Protection Unit/Zero Sequence Current ==
  Mag : Inport
  Phi : Inport  Port=2
  Add : Sum  Inputs=+++
  Complex to Magnitude-Angle : ComplexToMagnitudeAngle  Output=Magnitude
  Demux1 : Demux  Outputs=3
  Gain : Gain  Gain=1/3
  Magnitude-Angle to Complex : MagnitudeAngleToComplex
  I0 : Outport
  wires:
  Demux1/2 -> Add/2
  Demux1/3 -> Add/3
  Phi/1 -> Magnitude-Angle to Complex/2
  Complex to Magnitude-Angle/1 -> Gain/1
  Demux1/1 -> Add/1
  Mag/1 -> Magnitude-Angle to Complex/1
  Magnitude-Angle to Complex/1 -> Demux1/1
  Add/1 -> Complex to Magnitude-Angle/1
  Gain/1 -> I0/1

== system SP_OEL2/Relay2/Phase Protection Unit/Operating time  ==
  Current : Inport
  plugSetting : Inport  Port=2
  Constant : Constant  Value=phTimeSetting  VectorParams1D=off
  Constant3 : Constant  Value=relayCharacteristicPhase
  Constant9 : Constant  Value=relayCharacteristicPhase
  "Lookup table " : Subsystem
  MATLAB Function : MATLAB Function  TreatAsAtomicUnit=on
  Switch : Switch  Threshold=7  SaturateOnIntegerOverflow=off  InputSameDT=off
  Operating Time : Outport
  wires:
  Switch/1 -> Operating Time/1
  plugSetting/1 -> MATLAB Function/1(plugSetting)
  Constant9/1 -> Switch/2
  Constant/1 -> MATLAB Function/2(timeSetting)
  Constant3/1 -> MATLAB Function/3(relayCharacteristic)
  MATLAB Function/1(operatingTime) -> Switch/3
  "Lookup table "/1(Operating Time) -> Switch/1
  Current/1 -> "Lookup table "/1(Current)

== system SP_OEL2/Relay1/Earth Protection Unit/Operating Time/Lookup table ==
  Current : Inport
  2-D Lookup Table1 : Lookup_n-D  BreakpointsForDimension1=currentEarth  BreakpointsForDimension2=tmsEarth  Table=topEarth  InterpMethod=Cubic spline  ExtrapMethod=Cubic spline  InternalRulePriority=Speed  RndMeth=Simplest
      settings: InputPortMap=u0,u1
  Constant13 : Constant  Value=ethTimeSetting
  Constant16 : Constant  Value=topEarthActual
  Constant17 : Constant  Value=relayCharacteristicEarth
  Switch4 : Switch  Threshold=8  SaturateOnIntegerOverflow=off  InputSameDT=off
  Oeprating Time : Outport
  wires:
  Current/1 -> 2-D Lookup Table1/1
  Constant17/1 -> Switch4/2
  2-D Lookup Table1/1 -> Switch4/1
  Constant16/1 -> Switch4/3
  Constant13/1 -> 2-D Lookup Table1/2
  Switch4/1 -> Oeprating Time/1
